simulink model "Vehicle_Model_WIP_V3"  (R2019b)
settings: Solver=FixedStepDiscrete  StartTime=0.0  StopTime=Simulink.t_end  FixedStep=Simulink.dt  RelTol=1e-3
undefined symbols (not defined in the file): BRK, BTRRAD, CHLR, CHRG, DCDC, DiscIntNeverNeededParam, FAN, INV, MTR, PTRAD, PUMP, Settings, TRSM, Vehicle, VHCL, WHL
libraries: simulink x9, EV_cooling x6, EV_VLD x5, EV_ePWT x5
(part 4 of 5)

== system Vehicle_Model_WIP_V3/VLD/old/OLD VLD ==
  note: Vehicle Longitudinal Dynamic without slip model
  note: Vehicle Longitudinal Dynamic with slip model
  (0 == no)     (1 == yes) : Constant  Value=Simulink.slip
  Delay{6..11,13..14} (8 alike) : Delay  DelayLength=1
  Display : Display
  If : If  IfExpression=u1 == 0
  Merge{,1..9} (10 alike) : Merge
  Vehicle Longitudinal Dinamic  Model (No Slip) : Subsystem
  Vehicle Longitudinal Dinamic Model (Slip) : Subsystem
  l_km : Outport
  v_mps : Outport  Port=2
  a_mps2 : Outport  Port=3
  nWFr_RPM : Outport  Port=4
  vWFr_mps : Outport  Port=5
  nWRr_RPM : Outport  Port=6
  vWRr_mps : Outport  Port=7
  slipFr : Outport  Port=8
  slipRr : Outport  Port=9
  slipLoss_W : Outport  Port=10
  wires:
  Vehicle Longitudinal Dinamic  Model (No Slip)/4(VLD_nWhlFr_rpm) -> Merge3/1
  [VLD_mReal_kg] -> Vehicle Longitudinal Dinamic Model (Slip)/2(VLD_mReal_kg)
  Delay10/1 -> Vehicle Longitudinal Dinamic Model (Slip)/6(VLD_TWhlFrt_Nm)
  (0 == no)     (1 == yes)/1 -> If/1, Display/1
  Delay14/1 -> Vehicle Longitudinal Dinamic Model (Slip)/5(VLD_FRolRr_N)
  Delay11/1 -> Vehicle Longitudinal Dinamic Model (Slip)/7(VLD_TWhlRr_Nm)
  If/2 -> Vehicle Longitudinal Dinamic Model (Slip)/Action
  [VLD_MTotFrt_Nm] -> Delay10/1
  Merge4/1 -> vWFr_mps/1
  [INPT_vReq_kph] -> Vehicle Longitudinal Dinamic Model (Slip)/1(INPT_vReq_kph)
  Merge7/1 -> slipFr/1
  Vehicle Longitudinal Dinamic Model (Slip)/10(VLD_PTSlipLoss_W) -> Merge9/2
  Merge/1 -> l_km/1
  Vehicle Longitudinal Dinamic Model (Slip)/2(VLD_vActVhcl_mps) -> Merge1/2
  [VLD_MTotRr_Nm] -> Delay11/1
  Delay6/1 -> Vehicle Longitudinal Dinamic  Model (No Slip)/4(VLD_TWhlFrt_Nm)
  [VLD_WDisrtFr_N] -> Vehicle Longitudinal Dinamic Model (Slip)/8(VLD_WDisrtFr_N)
  Merge2/1 -> a_mps2/1
  Vehicle Longitudinal Dinamic  Model (No Slip)/1(VLD_lActVhcl_km) -> Merge/1
  [VLD_WDisrtRr_N] -> Vehicle Longitudinal Dinamic Model (Slip)/9(VLD_WDisrtRr_N)
  Vehicle Longitudinal Dinamic  Model (No Slip)/5(VLD_vWhlFr_mps) -> Merge4/1
  Vehicle Longitudinal Dinamic Model (Slip)/6(VLD_nWhlRr_rpm) -> Merge5/2
  Delay9/1 -> Vehicle Longitudinal Dinamic Model (Slip)/3(VLD_FRes_N)
  Delay7/1 -> Vehicle Longitudinal Dinamic  Model (No Slip)/3(VLD_FRst_N)
  [INPT_vReq_kph] -> Vehicle Longitudinal Dinamic  Model (No Slip)/1(INPT_vReq_kph)
  [VLD_mEquiv_kg] -> Vehicle Longitudinal Dinamic  Model (No Slip)/2(VLD_mEquiv_kg)
  Vehicle Longitudinal Dinamic  Model (No Slip)/2(VLD_vActVhcl_mps) -> Merge1/1
  Delay13/1 -> Vehicle Longitudinal Dinamic Model (Slip)/4(VLD_FRolFr_N)
  [VLD_FRolFr_N] -> Delay13/1
  Vehicle Longitudinal Dinamic  Model (No Slip)/7(VLD_vWhlRr_mps) -> Merge6/1
  Vehicle Longitudinal Dinamic  Model (No Slip)/9(VLD_rSlipRr) -> Merge8/1
  [VLD_RWhlRr_m] -> Vehicle Longitudinal Dinamic Model (Slip)/11(VLD_RWhlRr_m)
  [VLD_FRes_N] -> Delay9/1
  [VLD_RWhlFr_m] -> Vehicle Longitudinal Dinamic  Model (No Slip)/6(VLD_RWhlFr_m)
  If/1 -> Vehicle Longitudinal Dinamic  Model (No Slip)/Action
  [VLD_FRolRr_N] -> Delay14/1
  Merge6/1 -> vWRr_mps/1
  Vehicle Longitudinal Dinamic  Model (No Slip)/3(VLD_aActVhcl_mps2) -> Merge2/1
  Vehicle Longitudinal Dinamic Model (Slip)/9(VLD_rSlipRr) -> Merge8/2
  [VLD_RWhlRr_m] -> Vehicle Longitudinal Dinamic  Model (No Slip)/7(VLD_RWhlRr_m)
  [VLD_RWhlFr_m] -> Vehicle Longitudinal Dinamic Model (Slip)/10(VLD_RWhlFr_m)
  Vehicle Longitudinal Dinamic Model (Slip)/3(VLD_aActVhcl_mps2) -> Merge2/2
  [VLD_MTotFrt_Nm] -> Delay6/1
  Vehicle Longitudinal Dinamic Model (Slip)/7(VLD_vWhlRr_mps) -> Merge6/2
  [VLD_RrInrt_kgm2] -> Vehicle Longitudinal Dinamic Model (Slip)/13(VLD_RrInrt_kgm2)
  Vehicle Longitudinal Dinamic  Model (No Slip)/6(VLD_nWhlRr_rpm) -> Merge5/1
  [VLD_FRst_N] -> Delay7/1
  [VLD_MTotRr_Nm] -> Delay8/1
  Vehicle Longitudinal Dinamic  Model (No Slip)/10(VLD_PTSlipLoss_W) -> Merge9/1
  Delay8/1 -> Vehicle Longitudinal Dinamic  Model (No Slip)/5(VLD_TWhlRr_Nm)
  Merge8/1 -> slipRr/1
  Vehicle Longitudinal Dinamic  Model (No Slip)/8(VLD_rSlipFrt) -> Merge7/1
  [VLD_FrtInrt_kgm2] -> Vehicle Longitudinal Dinamic Model (Slip)/12(VLD_FrtInrt_kgm2)
  Merge1/1 -> v_mps/1
  Vehicle Longitudinal Dinamic Model (Slip)/1(VLD_lActVhcl_km) -> Merge/2
  Vehicle Longitudinal Dinamic Model (Slip)/5(VLD_vWhlFr_mps) -> Merge4/2
  Vehicle Longitudinal Dinamic Model (Slip)/4(VLD_nWhlFr_rpm) -> Merge3/2
  Vehicle Longitudinal Dinamic Model (Slip)/8(VLD_rSlipFrt) -> Merge7/2
  Merge3/1 -> nWFr_RPM/1
  Merge5/1 -> nWRr_RPM/1
  Merge9/1 -> slipLoss_W/1

== system Vehicle_Model_WIP_V3/VLD/old/Slope Force Calculation1 ==
  VLD_mReal_kg : Inport
  INPT_sReq_Pct : Inport  Port=2
  Atan : Trigonometry  Operator=atan
  Constant : Constant  Value=100
  Constant1 : Constant  Value=9.81
  Divide : Product  Inputs=*/
  Divide1 : Product
  Divide2 : Product
  Divide3 : Product
  Sin : Trigonometry
  Sin1 : Trigonometry  Operator=cos
  VLD_FSlp_N : Outport  VectorParamsAs1DForOutWhenUnconnected=off
  VLD_Wtot_N : Outport  Port=2  VectorParamsAs1DForOutWhenUnconnected=off
  wires:
  [VLD_Wtot_N] -> VLD_Wtot_N/1
  Divide3/1 -> [VLD_Wtot_N]
  Sin1/1 -> Divide3/2
  Divide2/1 -> [VLD_FSlp_N]
  Sin/1 -> Divide2/2
  Divide1/1 -> Divide2/1, Divide3/1
  Constant1/1 -> Divide1/2
  [VLD_mReal_kg] -> Divide1/1
  Atan/1 -> Sin/1, Sin1/1
  Divide/1 -> Atan/1
  Constant/1 -> Divide/2
  [INPT_sReq_Pct] -> Divide/1
  INPT_sReq_Pct/1 -> [INPT_sReq_Pct]
  VLD_mReal_kg/1 -> [VLD_mReal_kg]
  [VLD_FSlp_N] -> VLD_FSlp_N/1

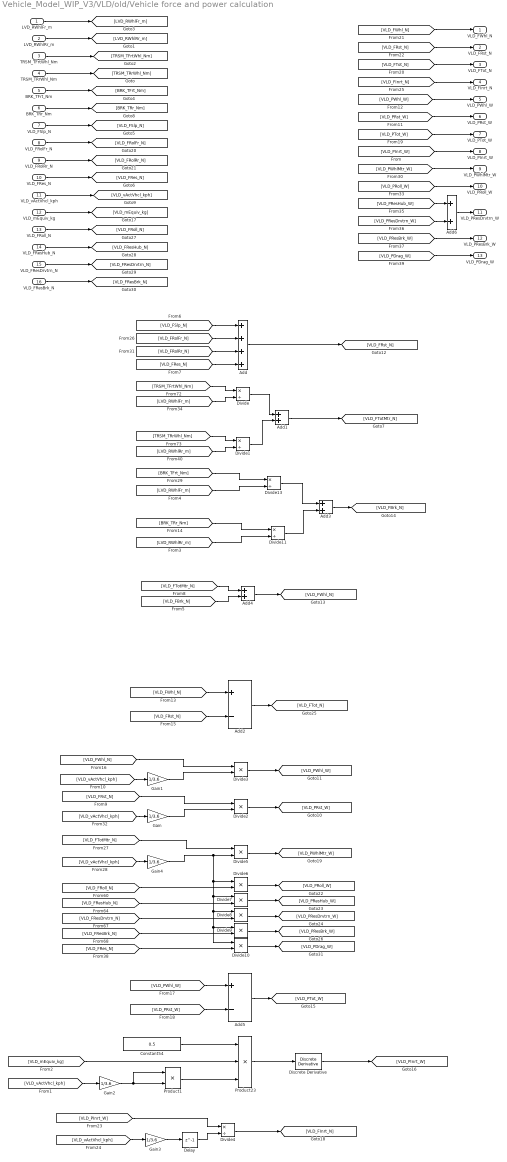
== system Vehicle_Model_WIP_V3/VLD/old/Vehicle force and power calculation ==
  LVD_RWhlFr_m : Inport
  LVD_RWhlRr_m : Inport  Port=2
  TRSM_TFrtWhl_Nm : Inport  Port=3
  TRSM_TRrWhl_Nm : Inport  Port=4
  BRK_TFrt_Nm : Inport  Port=5
  BRK_TRr_Nm : Inport  Port=6
  VLD_FSlp_N : Inport  Port=7
  VLD_FRolFr_N : Inport  Port=8
  VLD_FRolRr_N : Inport  Port=9
  VLD_FRes_N : Inport  Port=10
  VLD_vActVhcl_kph : Inport  Port=11
  VLD_mEquiv_kg : Inport  Port=12
  VLD_FRoll_N : Inport  Port=13
  VLD_FResHub_N : Inport  Port=14
  VLD_FResDrvtrn_N : Inport  Port=15
  VLD_FResBrk_N : Inport  Port=16
  Add : Sum  Inputs=++++
  Add{1,3..4,6} (4 alike) : Sum
  Add2 : Sum  Inputs=+-
  Add5 : Sum  Inputs=+-
  Constant54 : Constant  Value=0.5
  Delay : Delay  DelayLength=1  InitialCondition=1e-6
  Discrete Derivative : simulink/Discrete/Discrete Derivative  gainval=1.0  ICPrevScaledInput=0.0  OutMin=[]  OutMax=[]  OutDataType=fixdt(1, 16)  OutScaling=2^-10  DoSatur=off
  Divide{,1,4,11,13} (5 alike) : Product  Inputs=*/
  Divide{2..3,5..10} (8 alike) : Product
  Gain{,1..4} (5 alike) : Gain  Gain=1/3.6
  Product1 : Product  RndMeth=Zero
  Product23 : Product  Inputs=3  RndMeth=Zero
  VLD_FWhl_N : Outport  VectorParamsAs1DForOutWhenUnconnected=off
  VLD_FRst_N : Outport  Port=2  VectorParamsAs1DForOutWhenUnconnected=off
  VLD_FTot_N : Outport  Port=3  VectorParamsAs1DForOutWhenUnconnected=off
  VLD_FInrt_N : Outport  Port=4  VectorParamsAs1DForOutWhenUnconnected=off
  VLD_PWhl_W : Outport  Port=5  VectorParamsAs1DForOutWhenUnconnected=off
  VLD_PRst_W : Outport  Port=6  VectorParamsAs1DForOutWhenUnconnected=off
  VLD_PTot_W : Outport  Port=7  VectorParamsAs1DForOutWhenUnconnected=off
  VLD_PInrt_W : Outport  Port=8  VectorParamsAs1DForOutWhenUnconnected=off
  VLD_PWhlMtr_W : Outport  Port=9  VectorParamsAs1DForOutWhenUnconnected=off
  VLD_PRoll_W : Outport  Port=10  VectorParamsAs1DForOutWhenUnconnected=off
  VLD_PResDrvtrn_W : Outport  Port=11  VectorParamsAs1DForOutWhenUnconnected=off
  VLD_PResBrk_W : Outport  Port=12  VectorParamsAs1DForOutWhenUnconnected=off
  VLD_PDrag_W : Outport  Port=13  VectorParamsAs1DForOutWhenUnconnected=off
  wires:
  Add2/1 -> [VLD_FTot_N]
  [LVD_RWhlRr_m] -> Divide1/2
  Divide/1 -> Add1/1
  Divide1/1 -> Add1/2
  [TRSM_TRrWhl_Nm] -> Divide1/1
  Add1/1 -> [VLD_FTotMtr_N]
  TRSM_TRrWhl_Nm/1 -> [TRSM_TRrWhl_Nm]
  LVD_RWhlRr_m/1 -> [LVD_RWhlRr_m]
  LVD_RWhlFr_m/1 -> [LVD_RWhlFr_m]
  TRSM_TFrtWhl_Nm/1 -> [TRSM_TFrtWhl_Nm]
  [LVD_RWhlFr_m] -> Divide/2
  [TRSM_TFrtWhl_Nm] -> Divide/1
  BRK_TFrt_Nm/1 -> [BRK_TFrt_Nm]
  VLD_FSlp_N/1 -> [VLD_FSlp_N]
  VLD_FRes_N/1 -> [VLD_FRes_N]
  [VLD_FWhl_N] -> VLD_FWhl_N/1
  [VLD_FTot_N] -> VLD_FTot_N/1
  [LVD_RWhlRr_m] -> Divide11/2
  [LVD_RWhlFr_m] -> Divide13/2
  Divide13/1 -> Add3/1
  [BRK_TFrt_Nm] -> Divide13/1
  [BRK_TRr_Nm] -> Divide11/1
  Add3/1 -> [VLD_FBrk_N]
  Divide11/1 -> Add3/2
  BRK_TRr_Nm/1 -> [BRK_TRr_Nm]
  [VLD_FRst_N] -> VLD_FRst_N/1
  [VLD_vActVhcl_kph] -> Gain/1
  Add/1 -> [VLD_FRst_N]
  [VLD_FRes_N] -> Add/4
  [VLD_FSlp_N] -> Add/1
  Divide2/1 -> [VLD_PRst_W]
  Divide3/1 -> [VLD_PWhl_W]
  [VLD_FTotMtr_N] -> Add4/1
  [VLD_FBrk_N] -> Add4/2
  Add4/1 -> [VLD_FWhl_N]
  [VLD_vActVhcl_kph] -> Gain1/1
  [VLD_PWhl_W] -> VLD_PWhl_W/1
  [VLD_PRst_W] -> VLD_PRst_W/1
  [VLD_FRst_N] -> Divide2/1
  [VLD_FWhl_N] -> Divide3/1
  [VLD_FRst_N] -> Add2/2
  [VLD_FWhl_N] -> Add2/1
  [VLD_PWhl_W] -> Add5/1
  [VLD_PRst_W] -> Add5/2
  Add5/1 -> [VLD_PTot_W]
  [VLD_PTot_W] -> VLD_PTot_W/1
  Product1/1 -> Product23/3
  Constant54/1 -> Product23/1
  [VLD_mEquiv_kg] -> Product23/2
  Discrete Derivative/1 -> [VLD_PInrt_W]
  [VLD_vActVhcl_kph] -> Gain2/1
  Product23/1 -> Discrete Derivative/1
  VLD_mEquiv_kg/1 -> [VLD_mEquiv_kg]
  [VLD_PInrt_W] -> VLD_PInrt_W/1
  [VLD_PInrt_W] -> Divide4/1
  [VLD_vActVhcl_kph] -> Gain3/1
  Divide4/1 -> [VLD_FInrt_N]
  [VLD_FInrt_N] -> VLD_FInrt_N/1
  VLD_vActVhcl_kph/1 -> [VLD_vActVhcl_kph]
  Delay/1 -> Divide4/2
  Gain/1 -> Divide2/2
  Gain1/1 -> Divide3/2
  Gain2/1 -> Product1/1, Product1/2
  Gain3/1 -> Delay/1
  Gain4/1 -> Divide6/1, Divide10/1, Divide9/1, Divide8/1, Divide7/1, Divide5/2
  [VLD_vActVhcl_kph] -> Gain4/1
  [VLD_FTotMtr_N] -> Divide5/1
  Divide5/1 -> [VLD_PWhlMtr_W]
  [VLD_PWhlMtr_W] -> VLD_PWhlMtr_W/1
  VLD_FRolFr_N/1 -> [VLD_FRolFr_N]
  [VLD_FRolFr_N] -> Add/2
  VLD_FRolRr_N/1 -> [VLD_FRolRr_N]
  [VLD_FRolRr_N] -> Add/3
  [VLD_FRoll_N] -> Divide6/2
  [VLD_FResHub_N] -> Divide7/2
  [VLD_FResDrvtrn_N] -> Divide8/2
  [VLD_FResBrk_N] -> Divide9/2
  VLD_FResBrk_N/1 -> [VLD_FResBrk_N]
  VLD_FResDrvtrn_N/1 -> [VLD_FResDrvtrn_N]
  VLD_FResHub_N/1 -> [VLD_FResHub_N]
  VLD_FRoll_N/1 -> [VLD_FRoll_N]
  Divide6/1 -> [VLD_PRoll_W]
  Divide7/1 -> [VLD_PResHub_W]
  Divide8/1 -> [VLD_PResDrvtrn_W]
  Divide9/1 -> [VLD_PResBrk_W]
  [VLD_PRoll_W] -> VLD_PRoll_W/1
  [VLD_FRes_N] -> Divide10/2
  Divide10/1 -> [VLD_PDrag_W]
  [VLD_PResDrvtrn_W] -> Add6/2
  [VLD_PResHub_W] -> Add6/1
  Add6/1 -> VLD_PResDrvtrn_W/1
  [VLD_PResBrk_W] -> VLD_PResBrk_W/1
  [VLD_PDrag_W] -> VLD_PDrag_W/1

== system Vehicle_Model_WIP_V3/VLD/old/Weigth Distribution Front1 ==
  Mass real [kg] : Inport
  WTot_N : Inport  Port=2
  "Vehicle Actual Acc [m/s2] " : Inport  Port=3
  Vehicle Actual Speed [m/s] : Inport  Port=4
  Add1 : Sum  Inputs=+-
  Add2 : Sum  Inputs=+-
  Constant1 : Constant  Value=VHCL.Aero_surf
  Constant11 : Constant  Value=VHCL.Aero_Cl_Fr_HD
  Constant14 : Constant  Value=VHCL.Front_Weight_distrib_perc
  Constant15 : Constant  Value=VHCL.CG_height_m
  Constant16 : Constant  Value=VHCL.Wheelbase_mm
  Constant17 : Constant  Value=100
  Constant2 : Constant  Value=VHCL.Aero_Cl_Fr_LD
  Constant28 : Constant  Value=VHCL.Aero_WRS_kph
  Constant4 : Constant  Value=1000
  Display3 : Display
  Display4 : Display
  Display5 : Display
  Divide1 : Product  Inputs=****
  Divide13 : Product
  Divide17 : Product  Inputs=/*
  Divide18 : Product  Inputs=*/
  Divide2 : Product
  Divide3 : Product  Inputs=*/
  Divide4 : Product
  Gain : Gain
  Gain1 : Gain  Gain=3.6
  If Action Subsystem : Subsystem  TreatAsAtomicUnit=on
  If Action Subsystem1 : Subsystem  TreatAsAtomicUnit=on
  If1 : If  NumInputs=2  IfExpression=u1 < u2
  Merge : Merge
  Scope : Scope
  Scope9 : Scope
  Square : Math  Operator=square  SignedPower=off  SaturateOnIntegerOverflow=on
  density : Subsystem
  VLD_WDisrtFr_N : Outport  VectorParamsAs1DForOutWhenUnconnected=off
  wires:
  Gain1/1 -> If1/1
  Constant28/1 -> If1/2
  [Vehicle_Actual_Speed_mps] -> Gain1/1
  Constant2/1 -> If Action Subsystem1/1(In1)
  If Action Subsystem/1(Out1) -> Merge/2
  If Action Subsystem1/1(Out1) -> Merge/1
  Merge/1 -> Divide1/1
  Constant11/1 -> If Action Subsystem/1(In1)
  If1/1 -> If Action Subsystem1/Action
  If1/2 -> If Action Subsystem/Action
  Divide4/1 -> Add2/2
  Divide3/1 -> Divide4/2
  Divide2/1 -> Divide4/1
  Divide13/1 -> Add2/1
  [Vehicle_Actual_Acc_mps2] -> Divide2/2
  [Mass_Real_kg] -> Divide2/1
  Divide17/1 -> Divide13/1
  Constant17/1 -> Divide17/1
  Add1/1 -> Divide13/2
  Divide1/1 -> Add1/2, Scope/1
  [WTot_N] -> Add1/1
  Gain/1 -> Divide1/4
  Square/1 -> Divide1/3
  density/1(rho) -> Gain/1
  [Vehicle_Actual_Speed_mps] -> Square/1
  Constant1/1 -> Divide1/2
  WTot_N/1 -> [WTot_N]
  Constant14/1 -> Display5/1, Divide17/2
  Vehicle Actual Speed [m/s]/1 -> [Vehicle_Actual_Speed_mps]
  "Vehicle Actual Acc [m/s2] "/1 -> [Vehicle_Actual_Acc_mps2]
  Constant4/1 -> Divide18/2
  Constant15/1 -> Display3/1, Divide3/1
  Add2/1 -> [VLD_WDisrtFr_N], Scope9/1
  Divide18/1 -> Divide3/2
  Constant16/1 -> Display4/1, Divide18/1
  Mass real [kg]/1 -> [Mass_Real_kg]
  [VLD_WDisrtFr_N] -> VLD_WDisrtFr_N/1

== system Vehicle_Model_WIP_V3/VLD/old/Weigth Distribution Rear1 ==
  Mass real [kg] : Inport
  WTot_N : Inport  Port=2
  "Vehicle Actual Acc [m/s2] " : Inport  Port=3
  Vehicle Actual Speed [m/s] : Inport  Port=4
  Add1 : Sum  Inputs=+-
  Add2 : Sum
  Constant1 : Constant  Value=VHCL.Aero_surf
  Constant14 : Constant  Value=VHCL.Rear_Weight_distrib_perc
  Constant15 : Constant  Value=VHCL.CG_height_m
  Constant16 : Constant  Value=VHCL.Wheelbase_mm
  Constant17 : Constant  Value=100
  Constant2 : Constant  Value=VHCL.Aero_Cl_Rr_HD
  Constant28 : Constant  Value=VHCL.Aero_WRS_kph
  Constant3 : Constant  Value=VHCL.Aero_Cl_Rr_LD
  Constant4 : Constant  Value=1000
  Display3 : Display
  Display4 : Display
  Display5 : Display
  Divide1 : Product  Inputs=****
  Divide13 : Product
  Divide17 : Product  Inputs=/*
  Divide18 : Product  Inputs=*/
  Divide2 : Product
  Divide3 : Product  Inputs=*/
  Divide4 : Product
  Gain : Gain
  Gain1 : Gain  Gain=3.6
  If Action Subsystem : Subsystem  TreatAsAtomicUnit=on
  If Action Subsystem1 : Subsystem  TreatAsAtomicUnit=on
  If1 : If  NumInputs=2  IfExpression=u1 < u2
  Merge : Merge
  Scope : Scope
  Scope9 : Scope
  Square : Math  Operator=square  SignedPower=off  SaturateOnIntegerOverflow=on
  density : Subsystem
  VLD_WDisrtRr_N : Outport  VectorParamsAs1DForOutWhenUnconnected=off
  wires:
  [Vehicle_Actual_Speed_mps] -> Gain1/1
  Gain1/1 -> If1/1
  Constant28/1 -> If1/2
  If Action Subsystem1/1(Out1) -> Merge/1
  Merge/1 -> Divide1/1
  If1/1 -> If Action Subsystem1/Action
  If Action Subsystem/1(Out1) -> Merge/2
  Constant2/1 -> If Action Subsystem/1(In1)
  If1/2 -> If Action Subsystem/Action
  Constant3/1 -> If Action Subsystem1/1(In1)
  [VLD_WDisrtRr_N] -> VLD_WDisrtRr_N/1
  Mass real [kg]/1 -> [Mass_Real_kg]
  Constant16/1 -> Divide18/1, Display4/1
  Divide18/1 -> Divide3/2
  Add2/1 -> Scope9/1, [VLD_WDisrtRr_N]
  Constant15/1 -> Divide3/1, Display3/1
  Constant4/1 -> Divide18/2
  "Vehicle Actual Acc [m/s2] "/1 -> [Vehicle_Actual_Acc_mps2]
  Vehicle Actual Speed [m/s]/1 -> [Vehicle_Actual_Speed_mps]
  Constant14/1 -> Divide17/2, Display5/1
  WTot_N/1 -> [WTot_N]
  Constant1/1 -> Divide1/2
  [Vehicle_Actual_Speed_mps] -> Square/1
  density/1(rho) -> Gain/1
  Square/1 -> Divide1/3
  Gain/1 -> Divide1/4
  [WTot_N] -> Add1/1
  Divide1/1 -> Scope/1, Add1/2
  Add1/1 -> Divide13/2
  Constant17/1 -> Divide17/1
  Divide17/1 -> Divide13/1
  [Mass_Real_kg] -> Divide2/1
  [Vehicle_Actual_Acc_mps2] -> Divide2/2
  Divide13/1 -> Add2/1
  Divide2/1 -> Divide4/1
  Divide3/1 -> Divide4/2
  Divide4/1 -> Add2/2

== system Vehicle_Model_WIP_V3/old cooling/Battery Cooling system/Battery Pack Chiller ==
  RAD_TWtrOut_degC : Inport
  INIT_dVBtr_lpm : Inport  Port=2
  INIT_TSys_degC : Inport  Port=3
  VCU_bChlrEnbl : Inport  Port=4
  Constant : Constant  Value=0
  Constant3 : Constant  Value=CHLR.COP
  Delay : Delay  DelayLength=1  InitialConditionSource=Input port
      settings: InputPortMap=u0,p4
  "Density Water-Glycol 80-20%vol kg/m3 " : Lookup_n-D  NumberOfTableDimensions=1  BreakpointsForDimension1=[-45.56 -17.78 10 37.77 65.55 93.33 121.11 148.88 176.66]  Table=[1.02e+03 1.03e+03 1.03e+03 1.02e+03 9.99e+02 9.85e+02 9.63e+02 9.38e+02 9.11e+02]  ExtrapMethod=Clip  RndMeth=Simplest  InputSameDT=on
  Divide3 : Product
  Divide4 : Product  Inputs=*/
  Gain1 : Gain  Gain=1/60
  Gain2 : Gain  Gain=10^-3
  Heat Capacity  Water-Glycol 80-20%vol J/kgK : Lookup_n-D  NumberOfTableDimensions=1  BreakpointsForDimension1=[-45.56 -17.78 10 37.77 65.55 93.33 121.11 148.88 176.66]  Table="[3841.6 3888.1  3934.6 3981.1 4027.6 4074.0 4120.5 4167.0 4213.6]"  ExtrapMethod=Clip  RndMeth=Simplest  InputSameDT=on
  If : If  IfExpression=u1 == 1
  If Action Subsystem : Subsystem  TreatAsAtomicUnit=on
  If Action Subsystem1 : Subsystem  TreatAsAtomicUnit=on
  M vs V-n-t Motor Curve : Lookup_n-D  BreakpointsForDimension1=CHLR.dV_lpm_bp  BreakpointsForDimension2=CHLR.T_in_degC_bp  BreakpointsForDimension3=Vehicle.Motor.Front.bp_time  Table=CHLR.PCool_W  ExtrapMethod=Clip  UseLastTableValue=on  RndMeth=Simplest  InputSameDT=on
  Merge3 : Merge
  Mux : Mux  Inputs=2
  Product : Product
  Product1 : Product  Inputs=*/
  Product2 : Product
  Product3 : Product
  Scope : Scope  NumInputPorts=2
  Subsystem1 : Subsystem
  Subtract : Sum  Inputs=+-
  Subtract2 : Sum  Inputs=-+
  Terminator : Terminator
  CHLR_PHeatRej_W : Outport  VectorParamsAs1DForOutWhenUnconnected=off
  CHLR_TWtrOut_degC : Outport  Port=2  VectorParamsAs1DForOutWhenUnconnected=off
  CHLR_PElec_W : Outport  Port=3  VectorParamsAs1DForOutWhenUnconnected=off
  wires:
  [INIT_dVBtr_lpm] -> M vs V-n-t Motor Curve/1
  [CHLR_TWtrIn_degC] -> M vs V-n-t Motor Curve/2
  Subsystem1/1(Temp Water Bulk [°C]) -> Heat Capacity  Water-Glycol 80-20%vol J/kgK/1, "Density Water-Glycol 80-20%vol kg/m3 "/1
  [CHLR_TWtrIn_degC] -> Subsystem1/1(Temp Water Inlet [°C])
  "Density Water-Glycol 80-20%vol kg/m3 "/1 -> [CHLR_rhoCoolt_kgpm3]
  Heat Capacity  Water-Glycol 80-20%vol J/kgK/1 -> [CHLR_cpCoolt_JpkgK]
  [RAD_TWtrOut_degC] -> [CHLR_TWtrIn_degC]
  Constant3/1 -> Divide4/2
  [CHLR_PThrmCool_W] -> Divide4/1
  Divide4/1 -> [CHLR_PElec_W]
  INIT_TSys_degC/1 -> Terminator/1
  INIT_dVBtr_lpm/1 -> [INIT_dVBtr_lpm]
  RAD_TWtrOut_degC/1 -> [RAD_TWtrOut_degC]
  [CHLR_PElec_W] -> CHLR_PElec_W/1
  [CHLR_TWtrOut_degC] -> CHLR_TWtrOut_degC/1
  [CHLR_PHeatRej_W] -> CHLR_PHeatRej_W/1
  [INIT_dVBtr_lpm] -> Gain2/1
  Gain2/1 -> Divide3/1
  Divide3/1 -> Gain1/1
  [CHLR_rhoCoolt_kgpm3] -> Divide3/2
  Gain1/1 -> [CHLR_dmWtr_kgps]
  VCU_bChlrEnbl/1 -> [VCU_bChlrEnbl]
  If/1 -> If Action Subsystem/Action
  If Action Subsystem/1(Out1) -> Merge3/1
  If Action Subsystem1/1(Out1) -> Merge3/2
  If/2 -> If Action Subsystem1/Action
  M vs V-n-t Motor Curve/1 -> If Action Subsystem/1(In1)
  [VCU_bChlrEnbl] -> If/1
  Constant/1 -> If Action Subsystem1/1(In1)
  Merge3/1 -> Scope/2, [CHLR_PThrmCool_W]  "PThrmCool"
  Mux/1 -> Scope/1
  Subtract/1 -> Mux/2, [CHLR_TWtrOut_degC]  "TWtrOut"
  [CHLR_dmWtr_kgps] -> Product/1  "[kg/s]"
  [CHLR_cpCoolt_JpkgK] -> Product/2  "[J/kg/K]"
  Product/1 -> Product1/2
  [CHLR_PThrmCool_W] -> Product1/1
  [CHLR_TWtrIn_degC] -> Mux/1, Subtract/1  "TWtrIn"
  [CHLR_TWtrOut_degC] -> Subtract2/1
  [CHLR_TWtrIn_degC] -> Subtract2/2
  Product2/1 -> Product3/2
  [CHLR_cpCoolt_JpkgK] -> Product2/2  "[J/kg/K]"
  [CHLR_dmWtr_kgps] -> Product2/1  "[kg/s]"
  Subtract2/1 -> Product3/1
  Product3/1 -> [CHLR_PHeatRej_W]
  Product1/1 -> Subtract/2
  Delay/1 -> Subsystem1/2(Temp Water Outlet [°C])
  [CHLR_TWtrOut_degC] -> Delay/1
  [CHLR_TWtrIn_degC] -> Delay/2

== system Vehicle_Model_WIP_V3/old cooling/Battery Cooling system/Low Temperature Radiator ==
  BTR_TWtrOut_degC : Inport
  INIT_dVBtr_lpm : Inport  Port=2
  INPT_TEnv_degC : Inport  Port=3
  reset : Inport  Port=4
  RAD_dmAir_kgps : Inport  Port=5
  RAD_vAir_mps : Inport  Port=6
  Constant5 : Constant  Value=BTRRAD.AFrt_m2
  Density Water-Glycol 80-20%vol kg/m3 1 : Lookup_n-D  NumberOfTableDimensions=1  BreakpointsForDimension1=[-45.56 -17.78 10 37.77 65.55 93.33 121.11 148.88 176.66]  Table=[1.02e+03 1.03e+03 1.03e+03 1.02e+03 9.99e+02 9.85e+02 9.63e+02 9.38e+02 9.11e+02]  ExtrapMethod=Clip  RndMeth=Simplest  InputSameDT=on
  Divide8 : Product
  Divide9 : Product
  Gain1 : Gain  Gain=1/60
  Gain2 : Gain  Gain=10^-3
  M vs V-n-t Motor Curve1 : Lookup_n-D  BreakpointsForDimension1=BTRRAD.vAir_mps_bp  BreakpointsForDimension2=BTRRAD.dVWtr_lpm_bp  BreakpointsForDimension3=Vehicle.Motor.Front.bp_time  Table=BTRRAD.PHeatRej_Wpm2pK  ExtrapMethod=Clip  UseLastTableValue=on  RndMeth=Simplest  InputSameDT=on
  "Radiator Thermal model " : Subsystem
  Scope : Scope
  RAD_TWtrOut_degC : Outport  VectorParamsAs1DForOutWhenUnconnected=off
  RAD_PHeatRej_W : Outport  Port=2  VectorParamsAs1DForOutWhenUnconnected=off
  RAD_TAirOut_degC : Outport  Port=3  VectorParamsAs1DForOutWhenUnconnected=off
  wires:
  [RAD_dmWtr_kgps] -> "Radiator Thermal model "/4(RAD_dmWtr_kgps)
  [RAD_dmAir_kgps] -> "Radiator Thermal model "/3(RAD_dmAir_kgps)
  [RAD_TWtrIn_degC] -> "Radiator Thermal model "/2(RAD_TWtrIn_degC)
  [INPT_TEnv_degC] -> "Radiator Thermal model "/1(INPT_TEnv_degC)
  [RAD_UA_WpK] -> "Radiator Thermal model "/5(RAD_UA_WpK)
  [RAD_PHeatRej_W] -> RAD_PHeatRej_W/1
  INPT_TEnv_degC/1 -> [INPT_TEnv_degC]
  BTR_TWtrOut_degC/1 -> [BTR_TWtrOut_degC]
  INIT_dVBtr_lpm/1 -> [INIT_dVBtr_lpm]
  reset/1 -> [reset]
  Divide9/1 -> [RAD_UA_WpK]
  [INIT_dVBtr_lpm] -> M vs V-n-t Motor Curve1/2
  Constant5/1 -> Divide9/2
  Gain2/1 -> Divide8/1
  Gain1/1 -> [RAD_dmWtr_kgps]
  M vs V-n-t Motor Curve1/1 -> Scope/1, Divide9/1
  [RAD_vAir_mps] -> M vs V-n-t Motor Curve1/1
  [INIT_dVBtr_lpm] -> Gain2/1
  RAD_dmAir_kgps/1 -> [RAD_dmAir_kgps]
  Divide8/1 -> Gain1/1
  [RAD_rhoWtr] -> Divide8/2
  [BTR_TWtrOut_degC] -> [RAD_TWtrIn_degC]
  [RAD_TWtrOut_degC] -> RAD_TWtrOut_degC/1
  [RAD_TAirOut_degC] -> RAD_TAirOut_degC/1
  Density Water-Glycol 80-20%vol kg/m3 1/1 -> [RAD_rhoWtr]
  [RAD_TWtrBlk_degC] -> Density Water-Glycol 80-20%vol kg/m3 1/1
  RAD_vAir_mps/1 -> [RAD_vAir_mps]
  [reset] -> "Radiator Thermal model "/6(reset)
  "Radiator Thermal model "/4(RAD_PHeatRej_W) -> [RAD_PHeatRej_W]
  "Radiator Thermal model "/3(RAD_TWtrBlk_degC) -> [RAD_TWtrBlk_degC]
  "Radiator Thermal model "/2(RAD_TWtrOut_degC) -> [RAD_TWtrOut_degC]
  "Radiator Thermal model "/1(RAD_TAirOut_degC) -> [RAD_TAirOut_degC]

== system Vehicle_Model_WIP_V3/old cooling/Battery Cooling system/Pump Inertia ==
  VCU_dVBtr_lpm : Inport
  Discrete-Time Integrator : DiscreteIntegrator  InitialConditionSource=external  SampleTime=-1  ICPrevOutput=DiscIntNeverNeededParam  ICPrevScaledInput=DiscIntNeverNeededParam
  Divide6 : Product  Inputs=*/
  Divide7 : Product  Inputs=*/
  Divide8 : Product  Inputs=/*
  Subtract : Sum  Inputs=+-
  Tau : Constant  Value=3
  one : Constant
  BCS_dV_lpm : Outport
  wires:
  Discrete-Time Integrator/1 -> BCS_dV_lpm/1, Divide7/1
  Divide8/1 -> Divide6/2
  Tau/1 -> Divide7/2, Divide8/2
  VCU_dVBtr_lpm/1 -> Discrete-Time Integrator/2, Divide6/1
  one/1 -> Divide8/1
  Divide6/1 -> Subtract/1
  Subtract/1 -> Discrete-Time Integrator/1
  Divide7/1 -> Subtract/2

== system Vehicle_Model_WIP_V3/old cooling/Fan and air for Radiators/Air Flow and Fan Model ==
  note: Fan on-off
  note: Correction factor for the air velocity on the face af the radiator.
      | $\\ C = \frac{v_{vhcl}}{v_{rad}}$
  VLD_vActVhcl_kph : Inport
  INPT_TEnv_degC : Inport  Port=2
  VCU_bFanEnblPTCS : Inport  Port=3
  VCU_rFanFlow : Inport  Port=4
  Add : Sum
  AeroDynamic data for Radiator : Constant  Value=10
  Air Density kg/m : Lookup_n-D  NumberOfTableDimensions=1  BreakpointsForDimension1=[-40 -30 -20 -10 0 5 10 15 20 25 30 35 40 45 50 60 70 80 90 100]  Table=[1.514 1.451 1.394 1.341 1.292 1.269 1.246 1.225 1.204 1.184 1.164 1.145 1.127 1.109 1.092 1.059 1.028 0.9994 0.9718 0.9458]  ExtrapMethod=Clip  RndMeth=Simplest  InputSameDT=on
  Constant1 : Constant  Value=FAN.dVMx_m3ph
  Constant2 : Constant  Value=PTRAD.AFrt_m2
  Constant3 : Constant  Value=3.6
  Constant4 : Constant  Value=PTRAD.AFrt_m2
  Constant6 : Constant  Value=3600
  Divide : Product
  Divide1 : Product  Inputs=*//
  Divide10 : Product  Inputs=**/
  Divide5 : Product  Inputs=*/
  Divide6 : Product  Inputs=*/
  Divide7 : Product  Inputs=3
  Fan Inertia : Subsystem
  Fan Input Power [W] : Lookup_n-D  NumberOfTableDimensions=1  BreakpointsForDimension1=FAN.dV_bp  BreakpointsForDimension2=INV.Front.bp_Torque_Nm_Mtr  BreakpointsForDimension3=MTR.Front.bp_time  Table=FAN.Power  ExtrapMethod=Clip  UseLastTableValue=on  RndMeth=Simplest  InputSameDT=on
  If : If  IfExpression=u1 == 1
  If Action Subsystem : Subsystem  TreatAsAtomicUnit=on
  If Action Subsystem1 : Subsystem  TreatAsAtomicUnit=on
  Merge : Merge
  Zero : Constant  Value=0  OutDataTypeStr=Inherit: Inherit via back propagation
  RAD_dmAir_kgps : Outport
  RAD_VAirTot_mps : Outport  Port=2
  Fan_PwrReq_W : Outport  Port=3
  wires:
  Air Density kg/m/1 -> [RAD_rhoAir]
  Add/1 -> [RAD_dmAir_kgps]
  [VCU_rFanReqFlow] -> If Action Subsystem/1(In1)
  AeroDynamic data for Radiator/1 -> Divide6/2
  Constant4/1 -> Divide7/3
  [RAD_rhoAir] -> Divide10/2
  [VLD_vActVhcl_kph] -> Divide5/1
  Zero/1 -> If Action Subsystem1/1(In1)
  Fan Inertia/1(RAD_dVFan_m3ph) -> [RAD_dVFan_m3ph]
  Divide10/1 -> Add/2
  [RAD_dVFan_m3ph] -> Divide10/1
  Merge/1 -> Fan Inertia/1(Max Volumetric flow rate [lpm)
  [RAD_vAir_mps] -> Divide7/1
  Divide7/1 -> Add/1
  Divide5/1 -> Divide6/1
  [VCU_bFanEnblPTCS] -> If/1
  If/2 -> If Action Subsystem1/Action
  If Action Subsystem/1(Out1) -> Merge/1
  [RAD_rhoAir] -> Divide7/2
  If Action Subsystem1/1(Out1) -> Merge/2
  If/1 -> If Action Subsystem/Action
  Constant3/1 -> Divide5/2
  Divide6/1 -> [RAD_vAir_mps]
  Constant6/1 -> Divide10/3
  [INPT_TEnv_degC] -> Air Density kg/m/1
  VLD_vActVhcl_kph/1 -> [VLD_vActVhcl_kph]
  INPT_TEnv_degC/1 -> [INPT_TEnv_degC]
  VCU_bFanEnblPTCS/1 -> [VCU_bFanEnblPTCS]
  [RAD_dmAir_kgps] -> RAD_dmAir_kgps/1
  [RAD_dmAir_kgps] -> Divide1/1
  [RAD_rhoAir] -> Divide1/2
  Constant2/1 -> Divide1/3
  Divide1/1 -> [RAD_VAirTot_mps]
  [RAD_VAirTot_mps] -> RAD_VAirTot_mps/1
  VCU_rFanFlow/1 -> [VCU_rFanFlow]
  Constant1/1 -> Divide/1
  [VCU_rFanFlow] -> Divide/2
  Divide/1 -> [VCU_rFanReqFlow]
  Fan Input Power [W]/1 -> [Fan_PwrReq_W]
  [Fan_PwrReq_W] -> Fan_PwrReq_W/1
  [VCU_rFanReqFlow] -> Fan Input Power [W]/1

== system Vehicle_Model_WIP_V3/old cooling/PowerTrain Cooling system/Low Temperature Radiator ==
  MTR_TWtrOut_degC : Inport
  INIT_dVPwrT_lpm : Inport  Port=2
  RAD_dmAir_kgps : Inport  Port=3
  RADBCS_TAirOut_degC : Inport  Port=4
  RAD_vAir_mps : Inport  Port=5
  Constant2 : Constant  Value=PTRAD.AFrt_m2
  "Density Water-Glycol 80-20%vol kg/m3 " : Lookup_n-D  NumberOfTableDimensions=1  BreakpointsForDimension1=[-45.56 -17.78 10 37.77 65.55 93.33 121.11 148.88 176.66]  Table=[1.02e+03 1.03e+03 1.03e+03 1.02e+03 9.99e+02 9.85e+02 9.63e+02 9.38e+02 9.11e+02]  ExtrapMethod=Clip  RndMeth=Simplest  InputSameDT=on
  Divide3 : Product
  Divide4 : Product
  Gain3 : Gain  Gain=1/60
  Gain5 : Gain  Gain=10^-3
  M vs V-n-t Motor Curve : Lookup_n-D  BreakpointsForDimension1=PTRAD.vAir_mps_bp  BreakpointsForDimension2=PTRAD.dVWtr_lpm_bp  BreakpointsForDimension3=Vehicle.Motor.Front.bp_time  Table=PTRAD.PHeatRej_Wpm2pK  ExtrapMethod=Clip  UseLastTableValue=on  RndMeth=Simplest  InputSameDT=on
  "Radiator Thermal model " : Subsystem
  Scope : Scope
  Terminator : Terminator
  RAD_TWtrOut_degC : Outport  VectorParamsAs1DForOutWhenUnconnected=off
  RAD_PHeatRej_W : Outport  Port=2  VectorParamsAs1DForOutWhenUnconnected=off
  wires:
  [RAD_dmWtr_kgps] -> "Radiator Thermal model "/4(RAD_dmWtr_kgps)
  [RAD_dmAir_kgps] -> "Radiator Thermal model "/3(RAD_dmAir_kgps)
  [RAD_TWtrIn_degC] -> "Radiator Thermal model "/2(RAD_TWtrIn_degC)
  [RADBCS_TAirOut_degC] -> "Radiator Thermal model "/1(RADBCS_TAirOut_degC)
  [RAD_UA_WpK] -> "Radiator Thermal model "/5(RAD_UA_WpK)
  "Radiator Thermal model "/1(RAD_TAirOut_degC) -> Terminator/1
  "Radiator Thermal model "/2(RAD_TWtrOut_degC) -> [RAD_TWtrOut_degC]
  "Radiator Thermal model "/3(RAD_TWtrBlk_degC) -> [RAD_TWtrBlk_degC]
  [RAD_TWtrOut_degC] -> RAD_TWtrOut_degC/1
  [RAD_PHeatRej_W] -> RAD_PHeatRej_W/1
  "Radiator Thermal model "/4(RAD_PHeatRej_W) -> [RAD_PHeatRej_W]
  Gain3/1 -> [RAD_dmWtr_kgps]
  Gain5/1 -> Divide3/1
  Divide3/1 -> Gain3/1
  [INIT_dVPwrT_lpm] -> Gain5/1
  [RAD_rhoWtr] -> Divide3/2
  M vs V-n-t Motor Curve/1 -> Divide4/1
  [INIT_dVPwrT_lpm] -> M vs V-n-t Motor Curve/2
  [RAD_vAir_mps] -> M vs V-n-t Motor Curve/1
  Divide4/1 -> Scope/1, [RAD_UA_WpK]
  Constant2/1 -> Divide4/2
  MTR_TWtrOut_degC/1 -> [MTR_TWtrOut_degC]
  INIT_dVPwrT_lpm/1 -> [INIT_dVPwrT_lpm]
  "Density Water-Glycol 80-20%vol kg/m3 "/1 -> [RAD_rhoWtr]
  [RAD_TWtrBlk_degC] -> "Density Water-Glycol 80-20%vol kg/m3 "/1
  [MTR_TWtrOut_degC] -> [RAD_TWtrIn_degC]
  RAD_dmAir_kgps/1 -> [RAD_dmAir_kgps]
  RADBCS_TAirOut_degC/1 -> [RADBCS_TAirOut_degC]
  RAD_vAir_mps/1 -> [RAD_vAirTot_mps]
  [RAD_vAirTot_mps] -> [RAD_vAir_mps]

== system Vehicle_Model_WIP_V3/old cooling/PowerTrain Cooling system/Pump Inertia ==
  VCU_dVBtr_lpm : Inport
  Discrete-Time Integrator : DiscreteIntegrator  InitialConditionSource=external  SampleTime=-1  ICPrevOutput=DiscIntNeverNeededParam  ICPrevScaledInput=DiscIntNeverNeededParam
  Divide6 : Product  Inputs=*/
  Divide7 : Product  Inputs=*/
  Divide8 : Product  Inputs=/*
  Subtract : Sum  Inputs=+-
  Tau : Constant  Value=3
  one : Constant
  BCS_dV_lpm : Outport
  wires:
  Discrete-Time Integrator/1 -> BCS_dV_lpm/1, Divide7/1
  Divide8/1 -> Divide6/2
  Tau/1 -> Divide7/2, Divide8/2
  VCU_dVBtr_lpm/1 -> Discrete-Time Integrator/2, Divide6/1
  one/1 -> Divide8/1
  Divide6/1 -> Subtract/1
  Subtract/1 -> Discrete-Time Integrator/1
  Divide7/1 -> Subtract/2

== system Vehicle_Model_WIP_V3/VCU/Torque Distribution/TrqDistr/If Action Subsystem ==
  TCFr : Inport
  TCRr : Inport  Port=2
  Action Port : ActionPort  ActionPortLabel=else
  Fr : Outport
  Rr : Outport  Port=2
  wires:
  TCFr/1 -> Fr/1
  TCRr/1 -> Rr/1

== system Vehicle_Model_WIP_V3/VCU/Torque Distribution/TrqDistr/If Action Subsystem1 ==
  In1 : Inport
  In2 : Inport  Port=2
  Action Port : ActionPort  ActionPortLabel=if(u1 == 0)
  Out1 : Outport
  Out2 : Outport  Port=2
  wires:
  In2/1 -> Out2/1
  In1/1 -> Out1/1

== system Vehicle_Model_WIP_V3/VLD/old/OLD VLD/Vehicle Longitudinal Dinamic  Model (No Slip) ==
  note: Rear Wheels
  note: Front Wheels
  note: Slip Power Losses
  INPT_vReq_kph : Inport
  VLD_mEquiv_kg : Inport  Port=2
  VLD_FRst_N : Inport  Port=3
  VLD_TWhlFrt_Nm : Inport  Port=4
  VLD_TWhlRr_Nm : Inport  Port=5
  VLD_RWhlFr_m : Inport  Port=6
  VLD_RWhlRr_m : Inport  Port=7
  Action Port : ActionPort  ActionPortLabel=if(u1 == 0)
  Add : Sum  Inputs=+-
  Add1 : Sum
  Add2 : Sum  Inputs=+-
  Add3 : Sum  Inputs=+-
  Add4 : Sum
  Constant : Constant  Value=1e-6
  Constant1 : Constant  Value=0  VectorParams1D=off
  Constant6 : Constant  Value=0  VectorParams1D=off
  Discrete-Time Integrator : DiscreteIntegrator  InitialConditionSource=external  InitialCondition=1e-6  SampleTime=-1  LimitOutput=on  LowerSaturationLimit=1e-6  ICPrevOutput=DiscIntNeverNeededParam  ICPrevScaledInput=DiscIntNeverNeededParam
  Discrete-Time Integrator1 : DiscreteIntegrator  InitialCondition=1e-30  SampleTime=-1  ICPrevOutput=DiscIntNeverNeededParam  ICPrevScaledInput=DiscIntNeverNeededParam
  Divide : Product
  Divide{1..3,12,14} (5 alike) : Product  Inputs=*/
  Divide13 : Product  Inputs=**
  Divide15 : Product  Inputs=**
  Divide4 : Product
  Gain : Gain  Gain=3.6
  Gain1 : Gain  Gain=1e-3
  Gain3 : Gain  Gain=1/3.6
  Max : MinMax  Function=max  Inputs=2
  Wheel speed Front : Subsystem
  Wheel speed Rear : Subsystem
  VLD_lActVhcl_km : Outport
  VLD_vActVhcl_mps : Outport  Port=2
  VLD_aActVhcl_mps2 : Outport  Port=3
  VLD_nWhlFr_rpm : Outport  Port=4
  VLD_vWhlFr_mps : Outport  Port=5
  VLD_nWhlRr_rpm : Outport  Port=6
  VLD_vWhlRr_mps : Outport  Port=7
  VLD_rSlipFrt : Outport  Port=8
  VLD_rSlipRr : Outport  Port=9
  VLD_PTSlipLoss_W : Outport  Port=10
  wires:
  Divide13/1 -> Add4/1
  Divide4/1 -> [VLD_rSlipRr]
  Divide12/1 -> Divide13/2
  Wheel speed Front/1(VLD_nWhlFr_rpm) -> [VLD_nWhlFr_rpm]
  Wheel speed Front/2(VLD_vWhlFr_mps) -> [VLD_vWhlFr_mps]
  [VLD_RWhlFr_m] -> Divide12/2
  Wheel speed Rear/1(LVD_nWhlRr_rpm) -> [VLD_nWhlRr_rpm]
  [VLD_vActVhcl_mps] -> Add3/2
  [VLD_TWhlRr_Nm] -> Divide14/1
  Gain/1 -> [VLD_vActVhcl_kph]
  [VLD_vWhlRr_mps] -> VLD_vWhlRr_mps/1
  [VLD_TWhlRr_Nm] -> Divide3/1
  Gain1/1 -> [VLD_lActVhcl_km]
  [VLD_vWhlRr_mps] -> Add3/1
  [VLD_vActVhcl_mps] -> VLD_vActVhcl_mps/1
  Add/1 -> Divide2/1
  [VLD_TWhlFrt_Nm] -> Divide1/1
  Divide2/1 -> [VLD_aActVhcl_mps2], Discrete-Time Integrator/1
  [VLD_vActVhcl_kph] -> Wheel speed Rear/1(Vehicle Actual Speed [km/h])
  Discrete-Time Integrator/1 -> Gain/1, [VLD_vActVhcl_mps], Discrete-Time Integrator1/1
  Divide14/1 -> Divide15/2
  Divide1/1 -> Add1/1
  [VLD_RWhlFr_m] -> Divide1/2
  [VLD_RWhlRr_m] -> Wheel speed Rear/2(VLD_RWhlRr_m)
  Add1/1 -> Add/1
  [VLD_vActVhcl_kph] -> Wheel speed Front/1(Vehicle Actual Speed [km/h])
  [VLD_RWhlFr_m] -> Wheel speed Front/2(VLD_RWhlFr_m)
  Add3/1 -> Divide15/1
  [VLD_RWhlRr_m] -> Divide3/2
  [VLD_FRst_N] -> Add/2
  VLD_FRst_N/1 -> [VLD_FRst_N]
  Divide15/1 -> Add4/2
  [VLD_vActVhcl_mps] -> Add2/2
  [VLD_vWhlFr_mps] -> Add2/1
  Wheel speed Rear/2(VLD_vWhlRr_mps) -> [VLD_vWhlRr_mps]
  Divide3/1 -> Add1/2
  VLD_RWhlFr_m/1 -> [VLD_RWhlFr_m]
  [VLD_RWhlRr_m] -> Divide14/2
  Add4/1 -> [VLD_PTSlipLoss_W]
  Discrete-Time Integrator1/1 -> Gain1/1
  Add2/1 -> Divide13/1
  [VLD_aActVhcl_mps2] -> VLD_aActVhcl_mps2/1
  VLD_TWhlRr_Nm/1 -> [VLD_TWhlRr_Nm]
  VLD_RWhlRr_m/1 -> [VLD_RWhlRr_m]
  [VLD_lActVhcl_km] -> VLD_lActVhcl_km/1
  Max/1 -> Discrete-Time Integrator/2
  [VLD_vWhlFr_mps] -> VLD_vWhlFr_mps/1
  [VLD_nWhlRr_rpm] -> VLD_nWhlRr_rpm/1
  [VLD_nWhlFr_rpm] -> VLD_nWhlFr_rpm/1
  [VLD_PTSlipLoss_W] -> VLD_PTSlipLoss_W/1
  INPT_vReq_kph/1 -> [INPT_vReq_kph]
  Constant/1 -> Max/2
  VLD_TWhlFrt_Nm/1 -> [VLD_TWhlFrt_Nm]
  VLD_mEquiv_kg/1 -> [VLD_mEquiv_kg]
  Divide/1 -> [VLD_rSlipFrt]
  [VLD_mEquiv_kg] -> Divide2/2
  [VLD_TWhlFrt_Nm] -> Divide12/1
  [INPT_vReq_kph] -> Gain3/1
  Gain3/1 -> Max/1
  [VLD_rSlipFrt] -> VLD_rSlipFrt/1
  [VLD_rSlipRr] -> VLD_rSlipRr/1
  [VLD_vActVhcl_kph] -> Divide/1
  Constant6/1 -> Divide/2
  [VLD_vActVhcl_kph] -> Divide4/1
  Constant1/1 -> Divide4/2

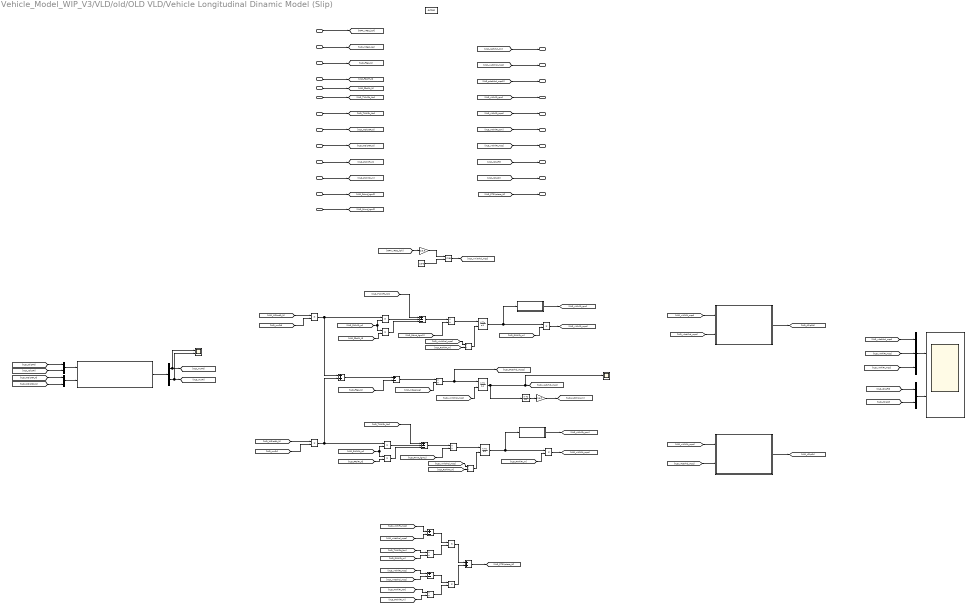
== system Vehicle_Model_WIP_V3/VLD/old/OLD VLD/Vehicle Longitudinal Dinamic Model (Slip) ==
  note: Slip Model
  note: Slip Power Losses
  note: Rear Wheels
  note: Front Wheels
  note: Tire Model
  note: Slip Model
  INPT_vReq_kph : Inport
  VLD_mReal_kg : Inport  Port=2
  VLD_FRes_N : Inport  Port=3
  VLD_FRolFr_N : Inport  Port=4
  VLD_FRolRr_N : Inport  Port=5
  VLD_TWhlFrt_Nm : Inport  Port=6
  VLD_TWhlRr_Nm : Inport  Port=7
  VLD_WDisrtFr_N : Inport  Port=8
  VLD_WDisrtRr_N : Inport  Port=9
  VLD_RWhlFr_m : Inport  Port=10
  VLD_RWhlRr_m : Inport  Port=11
  VLD_FrtInrt_kgm2 : Inport  Port=12
  VLD_RrInrt_kgm2 : Inport  Port=13
  Action Port : ActionPort  ActionPortLabel=else
  Add : Sum  Inputs=+-
  Add1 : Sum  Inputs=+-
  Add2 : Sum
  Add3 : Sum  Inputs=+--
  Add4 : Sum
  Add5 : Sum  Inputs=+-
  Add6 : Sum  Inputs=+--
  Constant : Constant  Value=1e-6
  Demux : Demux  Outputs=2
  Discrete-Time Integrator1 : DiscreteIntegrator  InitialCondition=1e-30  SampleTime=-1  ICPrevOutput=DiscIntNeverNeededParam  ICPrevScaledInput=DiscIntNeverNeededParam
  Discrete-Time Integrator2 : DiscreteIntegrator  InitialConditionSource=external  InitialCondition=30/0.37  SampleTime=-1  LimitOutput=on  LowerSaturationLimit=1e-6  ICPrevOutput=DiscIntNeverNeededParam  ICPrevScaledInput=DiscIntNeverNeededParam
  Discrete-Time Integrator3 : DiscreteIntegrator  InitialConditionSource=external  InitialCondition=30/0.37  SampleTime=-1  LimitOutput=on  LowerSaturationLimit=1e-6  ICPrevOutput=DiscIntNeverNeededParam  ICPrevScaledInput=DiscIntNeverNeededParam
  Discrete-Time Integrator4 : DiscreteIntegrator  InitialConditionSource=external  InitialCondition=30  SampleTime=-1  LimitOutput=on  LowerSaturationLimit=1e-6  ICPrevOutput=DiscIntNeverNeededParam  ICPrevScaledInput=DiscIntNeverNeededParam
  Divide{1,6,8..10,12,14} (7 alike) : Product  Inputs=*/
  Divide{2..5,7,11,13,15..17} (10 alike) : Product  Inputs=**
  Gain1 : Gain  Gain=1e-3
  Gain3 : Gain  Gain=1/3.6
  Max : MinMax  Function=max  Inputs=2
  Mux : Mux  Inputs=3
  Mux1 : Mux  Inputs=2
  Mux2 : Mux  Inputs=2
  Mux4 : Mux  Inputs=2
  Scope : Scope  NumInputPorts=2
  Scope1 : Scope
  Scope2 : Scope  NumInputPorts=2
  Slip Model Front : Subsystem
  Slip Model Rear : Subsystem
  Subsystem2 : Subsystem
  Subsystem3 : Subsystem
  Tire Model : Subsystem
  VLD_lActVhcl_km : Outport
  VLD_vActVhcl_mps : Outport  Port=2
  VLD_aActVhcl_mps2 : Outport  Port=3
  VLD_nWhlFr_rpm : Outport  Port=4
  VLD_vWhlFr_mps : Outport  Port=5
  VLD_nWhlRr_rpm : Outport  Port=6
  VLD_vWhlRr_mps : Outport  Port=7
  VLD_rSlipFrt : Outport  Port=8
  VLD_rSlipRr : Outport  Port=9
  VLD_PTSlipLoss_W : Outport  Port=10
  wires:
  [VLD_vActVhcl_mps] -> VLD_vActVhcl_mps/1
  [VLD_vWhlRr_mps] -> Slip Model Rear/1(VLD_vWhl_mps)
  [VLD_vActVhcl_mps] -> Slip Model Rear/2(VLD_vVhcl_mps)
  Slip Model Rear/1(slip) -> [VLD_rSlipRr]
  Slip Model Front/1(slip) -> [VLD_rSlipFrt]
  [VLD_vActVhcl_mps] -> Slip Model Front/2(VLD_vVhcl_mps)
  [VLD_vWhlFr_mps] -> Slip Model Front/1(VLD_vWhl_mps)
  Discrete-Time Integrator4/1 -> Discrete-Time Integrator1/1, [VLD_vActVhcl_mps], Scope1/1
  Add2/1 -> [VLD_PTSlipLoss_W]
  [VLD_rSlipFrt] -> VLD_rSlipFrt/1
  [VLD_rSlipRr] -> VLD_rSlipRr/1
  Gain1/1 -> [VLD_lActVhcl_km]
  Discrete-Time Integrator1/1 -> Gain1/1
  Divide16/1 -> Add6/2
  [VLD_RWhlRr_m] -> Divide17/2
  [VLD_rSlipRr] -> Mux4/2
  [VLD_RWhlRr_m] -> Divide2/1, Divide16/2
  [VLD_RWhlFr_m] -> Divide7/2
  VLD_RrInrt_kgm2/1 -> [VLD_RrInrt_kgm2]
  Max/1 -> [VLD_vInitVhcl_mps]
  [VLD_TWhlRr_Nm] -> Divide14/1
  VLD_mReal_kg/1 -> [VLD_mReal_kg]
  [VLD_lActVhcl_km] -> VLD_lActVhcl_km/1
  VLD_WDisrtFr_N/1 -> [VLD_WDisrtFr_N]
  Add5/1 -> Divide10/1
  Subsystem3/1(rpm) -> [VLD_nWhlRr_rpm]
  Tire Model/1(VLD_mu) -> Demux/1
  [VLD_mReal_kg] -> Divide10/2
  [VLD_WDisrtRr_N] -> Divide11/1
  VLD_RWhlFr_m/1 -> [VLD_RWhlFr_m]
  [VLD_muFrt] -> Divide4/2
  VLD_TWhlFrt_Nm/1 -> [VLD_TWhlFrt_Nm]
  [VLD_nWhlRr_rpm] -> VLD_nWhlRr_rpm/1
  Divide9/1 -> Discrete-Time Integrator3/1
  [VLD_WDisrtFr_N] -> Divide4/1
  Add4/1 -> Add5/1
  [VLD_FrtInrt_kgm2] -> Divide1/2
  Discrete-Time Integrator2/1 -> Subsystem2/1(rad/s), Divide7/1
  [VLD_PTSlipLoss_W] -> VLD_PTSlipLoss_W/1
  Add6/1 -> Divide9/1
  Add3/1 -> Divide1/1
  Divide12/1 -> Divide13/2
  Divide13/1 -> Add2/1
  Constant/1 -> Max/2
  [VLD_RWhlFr_m] -> Divide3/1, Divide5/2
  [VLD_vWhlRr_mps] -> VLD_vWhlRr_mps/1
  [VLD_rSlipFrt] -> Mux4/1
  Gain3/1 -> Max/1
  Demux/2 -> Scope2/2, [VLD_muRr]
  [VLD_vInitVhcl_mps] -> Discrete-Time Integrator4/2
  Divide7/1 -> [VLD_vWhlFr_mps]
  [INPT_vReq_kph] -> Gain3/1
  Demux/1 -> Scope2/1, [VLD_muFrt]
  Divide11/1 -> Divide16/1, Add4/2
  Divide14/1 -> Divide15/2
  Divide5/1 -> Add3/2
  INPT_vReq_kph/1 -> [INPT_vReq_kph]
  Subsystem2/1(rpm) -> [VLD_nWhlFr_rpm]
  [VLD_RWhlFr_m] -> Divide12/2
  VLD_FRes_N/1 -> [VLD_FRes_N]
  [VLD_vWhlFr_mps] -> Add/1
  Divide17/1 -> [VLD_vWhlRr_mps]
  Add1/1 -> Divide15/1
  Divide15/1 -> Add2/2
  [VLD_vActVhcl_mps] -> Add1/2
  VLD_FrtInrt_kgm2/1 -> [VLD_FrtInrt_kgm2]
  VLD_WDisrtRr_N/1 -> [VLD_WDisrtRr_N]
  VLD_RWhlRr_m/1 -> [VLD_RWhlRr_m]
  Divide4/1 -> Divide5/1, Add4/1
  VLD_TWhlRr_Nm/1 -> [VLD_TWhlRr_Nm]
  [VLD_vInitVhcl_mps] -> Divide8/1
  [VLD_nWhlFr_rpm] -> VLD_nWhlFr_rpm/1
  [VLD_aActVhcl_mps2] -> VLD_aActVhcl_mps2/1
  Mux4/1 -> Tire Model/1(VLD_rSlip)
  [VLD_vWhlRr_mps] -> Add1/1
  [VLD_vActVhcl_mps] -> Add/2
  [VLD_RrInrt_kgm2] -> Divide9/2
  Add/1 -> Divide13/1
  [VLD_muRr] -> Divide11/2
  Divide10/1 -> [VLD_aActVhcl_mps2], Discrete-Time Integrator4/1  "vdot"
  [VLD_vWhlFr_mps] -> VLD_vWhlFr_mps/1
  Discrete-Time Integrator3/1 -> Subsystem3/1(rad/s), Divide17/1
  [VLD_TWhlFrt_Nm] -> Divide12/1
  [VLD_RWhlRr_m] -> Divide14/2
  VLD_FRolFr_N/1 -> [VLD_FRolFr_N]
  [VLD_FRolFr_N] -> Divide3/2
  Mux/1 -> Scope/1
  [VLD_vWhlFr_mps] -> Mux/2
  [VLD_vWhlRr_mps] -> Mux/3
  [VLD_vActVhcl_mps] -> Mux/1
  Mux1/1 -> Scope/2
  [VLD_rSlipFrt] -> Mux1/1
  [VLD_rSlipRr] -> Mux1/2
  Divide3/1 -> Add3/3
  [VLD_FRolRr_N] -> Divide2/2
  [VLD_TWhlFrt_Nm] -> Add3/1
  [VLD_TWhlRr_Nm] -> Add6/1
  Divide1/1 -> Discrete-Time Integrator2/1
  [VLD_FRes_N] -> Add5/2
  [VLD_RWhlFr_m] -> Divide6/2
  [VLD_vInitVhcl_mps] -> Divide6/1
  Divide6/1 -> Discrete-Time Integrator2/2
  [VLD_RWhlRr_m] -> Divide8/2
  Divide8/1 -> Discrete-Time Integrator3/2
  VLD_FRolRr_N/1 -> [VLD_FRolRr_N]
  Divide2/1 -> Add6/3
  Mux2/1 -> Tire Model/2(VLD_WDistr)
  [VLD_WDisrtFr_N] -> Mux2/1
  [VLD_WDisrtRr_N] -> Mux2/2

== system Vehicle_Model_WIP_V3/VLD/old/Weigth Distribution Front1/If Action Subsystem ==
  In1 : Inport
  Action Port : ActionPort
  Out1 : Outport
  wires:
  In1/1 -> Out1/1

== system Vehicle_Model_WIP_V3/VLD/old/Weigth Distribution Front1/If Action Subsystem1 ==
  In1 : Inport
  Action Port : ActionPort
  Out1 : Outport
  wires:
  In1/1 -> Out1/1

== system Vehicle_Model_WIP_V3/VLD/old/Weigth Distribution Front1/density ==
  Constant : Constant  Value=273.15
  Constant1 : Constant  Value=Simulink.INIT_TEnv_degC
  Constant16 : Constant  Value=287
  Constant17 : Constant  Value=100000
  Divide10 : Product
  Divide11 : Product  Inputs=/*
  Subtract3 : Sum
  rho : Outport
  wires:
  Subtract3/1 -> Divide10/2
  Divide11/1 -> rho/1  "rho"
  Constant16/1 -> Divide10/1
  Constant1/1 -> Subtract3/1
  Constant17/1 -> Divide11/2  "p [Pa]"
  Constant/1 -> Subtract3/2
  Divide10/1 -> Divide11/1

== system Vehicle_Model_WIP_V3/VLD/old/Weigth Distribution Rear1/If Action Subsystem ==
  In1 : Inport
  Action Port : ActionPort
  Out1 : Outport
  wires:
  In1/1 -> Out1/1

== system Vehicle_Model_WIP_V3/VLD/old/Weigth Distribution Rear1/If Action Subsystem1 ==
  In1 : Inport
  Action Port : ActionPort
  Out1 : Outport
  wires:
  In1/1 -> Out1/1

== system Vehicle_Model_WIP_V3/VLD/old/Weigth Distribution Rear1/density ==
  Constant : Constant  Value=273.15
  Constant1 : Constant  Value=Simulink.INIT_TEnv_degC
  Constant16 : Constant  Value=287
  Constant17 : Constant  Value=100000
  Divide10 : Product
  Divide11 : Product  Inputs=/*
  Subtract3 : Sum
  rho : Outport
  wires:
  Divide10/1 -> Divide11/1
  Constant/1 -> Subtract3/2
  Constant17/1 -> Divide11/2  "p [Pa]"
  Constant1/1 -> Subtract3/1
  Constant16/1 -> Divide10/1
  Divide11/1 -> rho/1  "rho"
  Subtract3/1 -> Divide10/2

== system Vehicle_Model_WIP_V3/old cooling/Battery Cooling system/Battery Pack Chiller/If Action Subsystem ==
  In1 : Inport
  Action Port : ActionPort  ActionPortLabel=if(u1 == 1)
  Out1 : Outport
  wires:
  In1/1 -> Out1/1

== system Vehicle_Model_WIP_V3/old cooling/Battery Cooling system/Battery Pack Chiller/If Action Subsystem1 ==
  In1 : Inport
  Action Port : ActionPort  ActionPortLabel=else
  Out1 : Outport
  wires:
  In1/1 -> Out1/1

== system Vehicle_Model_WIP_V3/old cooling/Battery Cooling system/Battery Pack Chiller/Subsystem1 ==
  Temp Water Inlet [°C] : Inport
  Temp Water Outlet [°C] : Inport  Port=2
  Add1 : Sum  Inputs=+-
  Add9 : Sum
  Gain : Gain  Gain=1/2
  Mux3 : Mux  Inputs=3
  Scope3 : Scope
  Temp Water Bulk [°C] : Outport  VectorParamsAs1DForOutWhenUnconnected=off
  wires:
  Add9/1 -> Temp Water Bulk [°C]/1, Mux3/3  "T Bulk"
  Mux3/1 -> Scope3/1
  Temp Water Outlet [°C]/1 -> Add1/1, Mux3/1  "T Outlet"
  Temp Water Inlet [°C]/1 -> Add1/2, Add9/2, Mux3/2  "T Inlet"
  Add1/1 -> Gain/1
  Gain/1 -> Add9/1

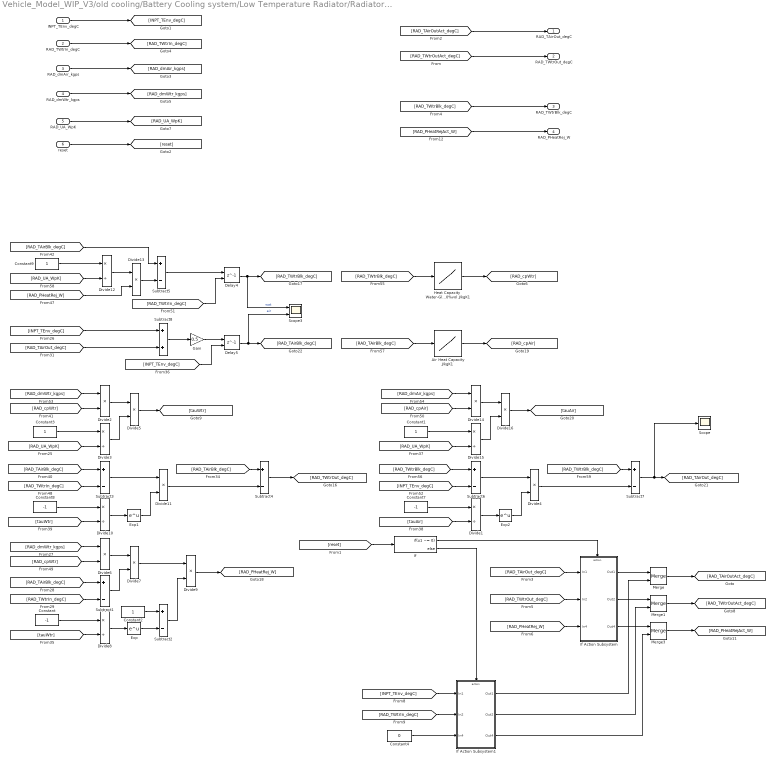
== system Vehicle_Model_WIP_V3/old cooling/Battery Cooling system/Low Temperature Radiator/Radiator Thermal model  ==
  INPT_TEnv_degC : Inport
  RAD_TWtrIn_degC : Inport  Port=2
  RAD_dmAir_kgps : Inport  Port=3
  RAD_dmWtr_kgps : Inport  Port=4
  RAD_UA_WpK : Inport  Port=5
  reset : Inport  Port=6
  Air Heat Capacity J/kgK1 : Lookup_n-D  NumberOfTableDimensions=1  BreakpointsForDimension1=[-40 -30 -20 -10 0 5 10 15 20 25 30 35 40 45 50 60 70 80 90 100]  Table=[1002 1004 1005 1006 1006 1007 1008 1009 1010 1011 1011 1012 1013 1014 1016 1017 1019 1020 1021 1022]  ExtrapMethod=Clip  RndMeth=Simplest  InputSameDT=on
  Constant : Constant  Value=-1
  Constant{1..3,9} (4 alike) : Constant
  Constant4 : Constant  Value=0
  Constant7 : Constant  Value=-1
  Constant8 : Constant  Value=-1
  Delay4 : Delay  DelayLength=1  InitialConditionSource=Input port
      settings: InputPortMap=u0,p4
  Delay5 : Delay  DelayLength=1  InitialConditionSource=Input port
      settings: InputPortMap=u0,p4
  Divide{1,3,8,10,12,15} (6 alike) : Product  Inputs=*/
  Divide{2,4..7,9,11,13..14,16} (10 alike) : Product  Inputs=**
  Exp : Math  SignedPower=off  SaturateOnIntegerOverflow=on
  Exp1 : Math  SignedPower=off  SaturateOnIntegerOverflow=on
  Exp2 : Math  SignedPower=off  SaturateOnIntegerOverflow=on
  Gain : Gain  Gain=0.5
  Heat Capacity  Water-Glycol 80-20%vol J/kgK1 : Lookup_n-D  NumberOfTableDimensions=1  BreakpointsForDimension1=[-45.56 -17.78 10 37.77 65.55 93.33 121.11 148.88 176.66]  Table="[3841.6 3888.1  3934.6 3981.1 4027.6 4074.0 4120.5 4167.0 4213.6]"  ExtrapMethod=Clip  RndMeth=Simplest  InputSameDT=on
  If : If  IfExpression=u1 ~= 0
  If Action Subsystem : Subsystem  TreatAsAtomicUnit=on
  If Action Subsystem1 : Subsystem  TreatAsAtomicUnit=on
  Merge : Merge
  Merge1 : Merge
  Merge3 : Merge
  Scope : Scope
  Scope3 : Scope  NumInputPorts=2
  Subtract{1..7} (7 alike) : Sum  Inputs=+-
  Subtract8 : Sum
  RAD_TAirOut_degC : Outport  VectorParamsAs1DForOutWhenUnconnected=off
  RAD_TWtrOut_degC : Outport  Port=2  VectorParamsAs1DForOutWhenUnconnected=off
  RAD_TWtrBlk_degC : Outport  Port=3  VectorParamsAs1DForOutWhenUnconnected=off
  RAD_PHeatRej_W : Outport  Port=4  VectorParamsAs1DForOutWhenUnconnected=off
  wires:
  [RAD_TWtrBlk_degC] -> RAD_TWtrBlk_degC/1
  [RAD_TAirOutAct_degC] -> RAD_TAirOut_degC/1
  [RAD_TWtrOutAct_degC] -> RAD_TWtrOut_degC/1
  [RAD_PHeatRejAct_W] -> RAD_PHeatRej_W/1
  INPT_TEnv_degC/1 -> [INPT_TEnv_degC]
  RAD_TWtrIn_degC/1 -> [RAD_TWtrIn_degC]
  RAD_UA_WpK/1 -> [RAD_UA_WpK]
  RAD_dmAir_kgps/1 -> [RAD_dmAir_kgps]
  RAD_dmWtr_kgps/1 -> [RAD_dmWtr_kgps]
  [INPT_TEnv_degC] -> Subtract8/1
  Gain/1 -> Delay5/1
  Subtract7/1 -> Scope/1, [RAD_TAirOut_degC]
  Subtract8/1 -> Gain/1
  [RAD_TAirOut_degC] -> Subtract8/2
  Heat Capacity  Water-Glycol 80-20%vol J/kgK1/1 -> [RAD_cpWtr]
  [RAD_TAirBlk_degC] -> Air Heat Capacity J/kgK1/1
  [RAD_dmWtr_kgps] -> Divide6/1
  Divide4/1 -> Subtract7/2
  [RAD_cpAir] -> Divide14/2
  [RAD_UA_WpK] -> Divide15/2
  [RAD_TAirBlk_degC] -> Subtract4/1
  Divide14/1 -> Divide16/1
  Exp2/1 -> Divide4/2
  [RAD_cpWtr] -> Divide6/2
  Constant9/1 -> Divide12/1
  Delay4/1 -> Scope3/1, [RAD_TWtrBlk_degC]  "wat"
  [RAD_TWtrBlk_degC] -> Heat Capacity  Water-Glycol 80-20%vol J/kgK1/1
  Constant3/1 -> Divide3/1
  [RAD_TWtrBlk_degC] -> Subtract6/1
  Subtract4/1 -> [RAD_TWtrOut_degC]
  [RAD_TAirBlk_degC] -> Subtract1/1
  [tauWtr] -> Divide10/2
  Constant2/1 -> Subtract2/1
  Subtract1/1 -> Divide7/2
  Divide5/1 -> [tauWtr]
  Divide13/1 -> Subtract5/2
  [INPT_TEnv_degC] -> Subtract6/2
  Subtract3/1 -> Divide11/1
  Constant8/1 -> Divide10/1
  Exp/1 -> Subtract2/2
  Divide9/1 -> [RAD_PHeatRej_W]
  [RAD_dmAir_kgps] -> Divide14/1
  [RAD_PHeatRej_W] -> Divide13/2
  Delay5/1 -> Scope3/2, [RAD_TAirBlk_degC]  "air"
  [RAD_TWtrBlk_degC] -> Subtract7/1
  Divide6/1 -> Divide7/1
  Divide7/1 -> Divide9/1
  Divide1/1 -> Exp2/1
  Constant/1 -> Divide8/1
  Divide8/1 -> Exp/1
  [INPT_TEnv_degC] -> Delay5/2
  Subtract2/1 -> Divide9/2
  Divide10/1 -> Exp1/1
  Subtract6/1 -> Divide4/1
  Divide12/1 -> Divide13/1
  [RAD_TWtrIn_degC] -> Subtract3/2
  [RAD_TWtrIn_degC] -> Delay4/2
  Divide2/1 -> Divide5/1
  Exp1/1 -> Divide11/2
  [RAD_dmWtr_kgps] -> Divide2/1
  Divide15/1 -> Divide16/2
  [RAD_UA_WpK] -> Divide12/2
  [RAD_TAirBlk_degC] -> Subtract5/1
  Subtract5/1 -> Delay4/1
  Constant1/1 -> Divide15/1
  [RAD_cpWtr] -> Divide2/2
  Divide3/1 -> Divide5/2
  Air Heat Capacity J/kgK1/1 -> [RAD_cpAir]
  [RAD_TWtrIn_degC] -> Subtract1/2
  [tauAir] -> Divide1/2
  [tauWtr] -> Divide8/2
  Constant7/1 -> Divide1/1
  Divide11/1 -> Subtract4/2
  Divide16/1 -> [tauAir]
  [RAD_UA_WpK] -> Divide3/2
  [RAD_TAirBlk_degC] -> Subtract3/1
  reset/1 -> [reset]
  [reset] -> If/1
  If/1 -> If Action Subsystem/Action
  If/2 -> If Action Subsystem1/Action
  [RAD_TAirOut_degC] -> If Action Subsystem/1(In1)
  If Action Subsystem/1(Out1) -> Merge/1
  If Action Subsystem/2(Out2) -> Merge1/1
  Merge1/1 -> [RAD_TWtrOutAct_degC]
  If Action Subsystem/3(Out4) -> Merge3/1
  Merge3/1 -> [RAD_PHeatRejAct_W]
  Merge/1 -> [RAD_TAirOutAct_degC]
  If Action Subsystem1/1(Out1) -> Merge/2
  If Action Subsystem1/2(Out2) -> Merge1/2
  If Action Subsystem1/3(Out4) -> Merge3/2
  [RAD_TWtrOut_degC] -> If Action Subsystem/2(In2)
  [RAD_PHeatRej_W] -> If Action Subsystem/3(In4)
  [INPT_TEnv_degC] -> If Action Subsystem1/1(In1)
  [RAD_TWtrIn_degC] -> If Action Subsystem1/2(In2)
  Constant4/1 -> If Action Subsystem1/3(In4)
